simulink model "validity"  (R2021b)
settings: Solver=FixedStepAuto  StartTime=0.0  StopTime=10.0  RelTol=1e-3
undefined symbols (not defined in the file): DiscIntNeverNeededParam, sldvsubsys
libraries: sldvlib x8
settings Model: Creator=marco  LastModifiedBy=angelo
settings ConfigComp: DVMode=PropertyProving  DVMaxProcessTime=14400  DVTestSuiteOptimization=Auto  DVDetectOutOfBounds=on  DVMaxViolationSteps=5  DVModelReferenceHarness=on

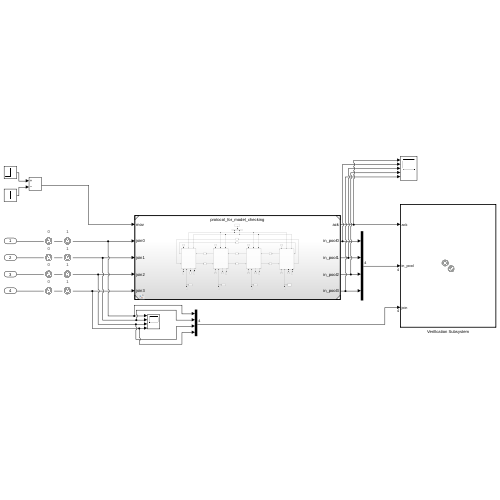
[thumbnail: Simulink's stored preview of the top-level diagram]
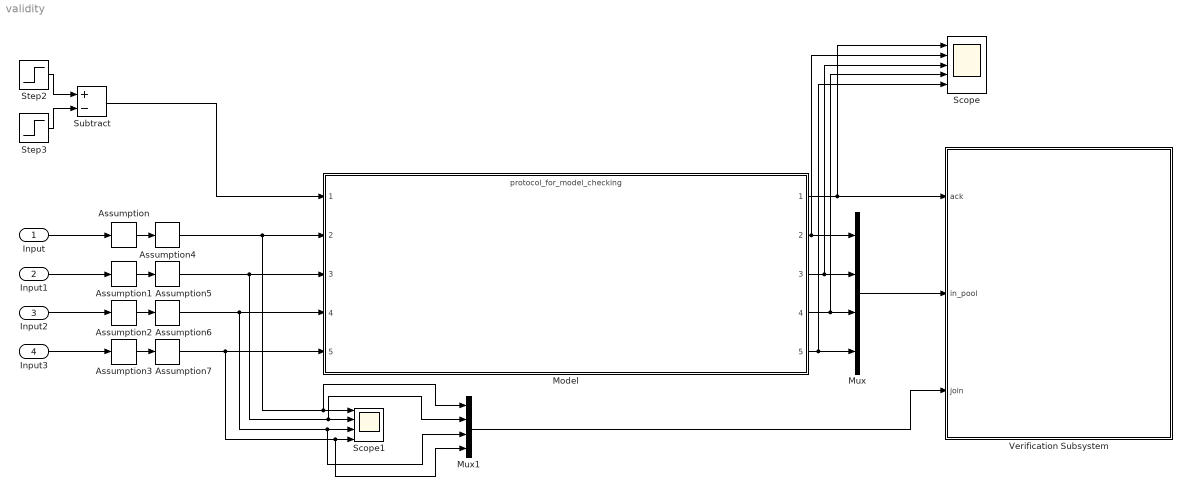
== system validity ==
  Input : Inport
  Input1 : Inport  Port=2
  Input2 : Inport  Port=3
  Input3 : Inport  Port=4
  Assumption{,1..3} (4 alike) : sldvlib/Objectives and Constraints/Assumption  enabled=on  customAVTBlockType=Assumption  intervals=0  initial=off  dispValues=on  outEnabled=on
      settings: AttributesFormatString=%<intervals>  SourceProductBaseCode=SL
  Assumption{4..7} (4 alike) : sldvlib/Objectives and Constraints/Assumption  enabled=on  customAVTBlockType=Assumption  intervals=1  initial=off  dispValues=on  outEnabled=on
      settings: AttributesFormatString=%<intervals>  SourceProductBaseCode=SL
  Model : ModelReference  ModelNameDialog=protocol_for_model_checking.slx  SimulationMode=Normal  ModelReferenceVersion=1.102
  Mux : Mux
  Mux1 : Mux
  Scope : Scope  NumInputPorts=5
  Scope1 : Scope  NumInputPorts=4
  Step2 : Step  SampleTime=.2
  Step3 : Step  Time=1.2  SampleTime=.2
  Subtract : Sum  Inputs=+-
  Verification Subsystem : Subsystem  Tag=VerificationSubsystem  DisableCoverage=on  LoadFcn=sldvsubsys('check')  TreatAsAtomicUnit=on  SimViewingDevice=on  mask(VerificationSubsystem){}
      mask init:
      | sldvsubsys('maskInit');
      settings: CopyFcn=sldvsubsys('copy');  OpenFcn=open_system(gcb,'force');
      settings: PreSaveFcn=|
      | set_param(gcb,'SimViewingDevice','on');
      | sldvsubsys('check');
      mask Help: helpview(fullfile(docroot,'toolbox','sldv','sldv.map'),'verificationsubsystem')
      mask Display: image(imread('sldvicon_versubsys.png','BackGroundColor',[1 1 1]),'center');
  wires:
  Mux/1 -> Verification Subsystem/2(in_pool)
  Step3/1 -> Subtract/2
  Step2/1 -> Subtract/1
  Subtract/1 -> Model/1
  Model/2 -> Scope/2, Mux/1
  Model/3 -> Scope/3, Mux/2
  Model/4 -> Scope/4, Mux/3
  Model/5 -> Scope/5, Mux/4
  Model/1 -> Scope/1, Verification Subsystem/1(ack)
  Assumption/1 -> Assumption4/1
  Assumption1/1 -> Assumption5/1
  Assumption2/1 -> Assumption6/1
  Assumption3/1 -> Assumption7/1
  Input/1 -> Assumption/1
  Input1/1 -> Assumption1/1
  Input2/1 -> Assumption2/1
  Input3/1 -> Assumption3/1
  Mux1/1 -> Verification Subsystem/3(join)
  Assumption4/1 -> Mux1/1, Scope1/1, Model/2
  Assumption5/1 -> Mux1/2, Scope1/2, Model/3
  Assumption6/1 -> Mux1/3, Scope1/3, Model/4
  Assumption7/1 -> Mux1/4, Scope1/4, Model/5

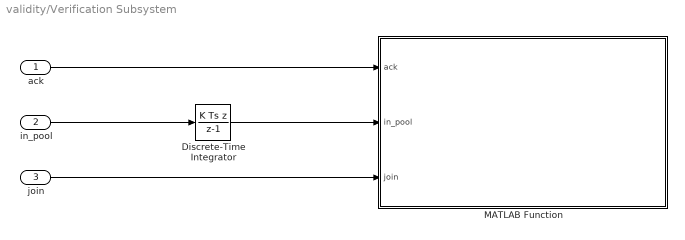
== system validity/Verification Subsystem ==
  ack : Inport
  in_pool : Inport  Port=2
  join : Inport  Port=3
  Discrete-Time Integrator : DiscreteIntegrator  IntegratorMethod=Integration: Backward Euler  SampleTime=-1  ICPrevOutput=DiscIntNeverNeededParam  ICPrevScaledInput=DiscIntNeverNeededParam
  MATLAB Function : MATLAB Function  TreatAsAtomicUnit=on
  wires:
  join/1 -> MATLAB Function/3(join)
  in_pool/1 -> Discrete-Time Integrator/1
  Discrete-Time Integrator/1 -> MATLAB Function/2(in_pool)
  ack/1 -> MATLAB Function/1(ack)

== matlab function validity/Verification Subsystem/MATLAB Function ==
  data: ack input; in_pool input; join input
function validity(ack, in_pool, join)
    if(ack > 0)
        in_pool = in_pool > 0;
        sldv.prove(all((in_pool & join) == in_pool));
    end
end
